simulink model "simu_first_circuit_paper"  (Simulink 7.5)
settings: Solver=ode45  StartTime=0.0  StopTime=10.0  RelTol=1e-3
values from neighbouring files (symbols this model uses):
  b1 = 500    [initialise_parameters.m]
  b2 = 1500    [initialise_parameters.m]
  k1 = 60000*4    (= 240000)    [initialise_parameters.m]
  k2 = 1350000*4    (= 5400000)    [initialise_parameters.m]
  m1 = 500    [initialise_parameters.m]
  m2 = 50    [initialise_parameters.m]
settings Model: Creator=Arijit  LastModifiedBy=Arijit

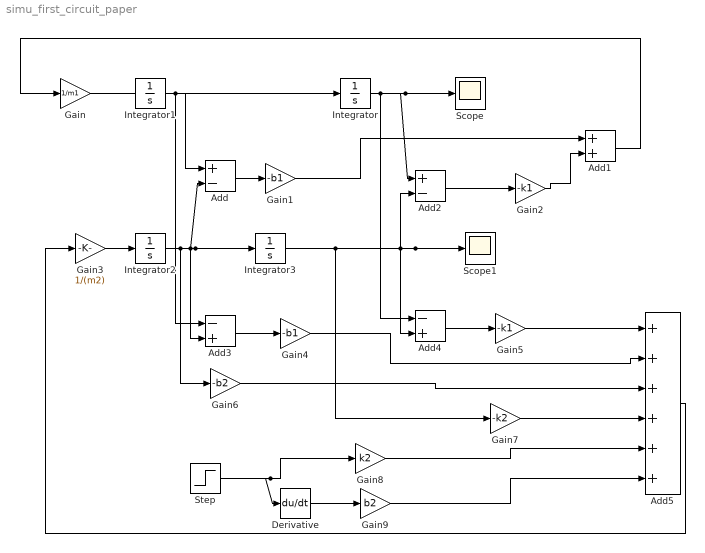
== system simu_first_circuit_paper ==
  Add : Sum  Inputs=+-  OutDataType=fixdt(1, 16)  OutScaling=2^-10
  Add1 : Sum  OutDataType=fixdt(1, 16)  OutScaling=2^-10
  Add2 : Sum  Inputs=+-  OutDataType=fixdt(1, 16)  OutScaling=2^-10
  Add3 : Sum  Inputs=-+  OutDataType=fixdt(1, 16)  OutScaling=2^-10
  Add4 : Sum  Inputs=-+  OutDataType=fixdt(1, 16)  OutScaling=2^-10
  Add5 : Sum  Inputs=++++++  OutDataType=fixdt(1, 16)  OutScaling=2^-10
  Derivative : Derivative
  Gain : Gain  Gain=1/m1  ParameterDataType=fixdt(1, 16)  ParameterScaling=2^0  OutDataType=fixdt(1, 16)  OutScaling=2^0
  Gain1 : Gain  Gain=-b1  ParameterDataType=fixdt(1, 16)  ParameterScaling=2^0  OutDataType=fixdt(1, 16)  OutScaling=2^0
  Gain2 : Gain  Gain=-k1  ParameterDataType=fixdt(1, 16)  ParameterScaling=2^0  OutDataType=fixdt(1, 16)  OutScaling=2^0
  Gain3 : Gain  Gain=1/(m2)  ParameterDataType=fixdt(1, 16)  ParameterScaling=2^0  OutDataType=fixdt(1, 16)  OutScaling=2^0
  Gain4 : Gain  Gain=-b1  ParameterDataType=fixdt(1, 16)  ParameterScaling=2^0  OutDataType=fixdt(1, 16)  OutScaling=2^0
  Gain5 : Gain  Gain=-k1  ParameterDataType=fixdt(1, 16)  ParameterScaling=2^0  OutDataType=fixdt(1, 16)  OutScaling=2^0
  Gain6 : Gain  Gain=-b2  ParameterDataType=fixdt(1, 16)  ParameterScaling=2^0  OutDataType=fixdt(1, 16)  OutScaling=2^0
  Gain7 : Gain  Gain=-k2  ParameterDataType=fixdt(1, 16)  ParameterScaling=2^0  OutDataType=fixdt(1, 16)  OutScaling=2^0
  Gain8 : Gain  Gain=k2  ParameterDataType=fixdt(1, 16)  ParameterScaling=2^0  OutDataType=fixdt(1, 16)  OutScaling=2^0
  Gain9 : Gain  Gain=b2  ParameterDataType=fixdt(1, 16)  ParameterScaling=2^0  OutDataType=fixdt(1, 16)  OutScaling=2^0
  Integrator{,1..3} (4 alike) : Integrator
  Scope : Scope
  Scope1 : Scope
  Step : Step  SampleTime=0
  wires:
  Gain/1 -> Integrator1/1, Add/1, Add3/1
  Integrator1/1 -> Integrator/1
  Integrator/1 -> Scope/1, Add2/1, Add4/1
  Add/1 -> Gain1/1
  Gain1/1 -> Add1/1
  Add1/1 -> Gain/1
  Add2/1 -> Gain2/1
  Gain2/1 -> Add1/2
  Gain3/1 -> Integrator2/1
  Integrator2/1 -> Add3/2, Integrator3/1, Add/2, Gain6/1
  Integrator3/1 -> Scope1/1, Add2/2, Add4/2, Gain7/1
  Add3/1 -> Gain4/1
  Add4/1 -> Gain5/1
  Gain5/1 -> Add5/1
  Gain4/1 -> Add5/2
  Gain6/1 -> Add5/3
  Gain7/1 -> Add5/4
  Step/1 -> Gain8/1, Derivative/1
  Derivative/1 -> Gain9/1
  Gain9/1 -> Add5/6
  Gain8/1 -> Add5/5
  Add5/1 -> Gain3/1
